simulink model "javelinSimplified"  (R2025b)
settings: Solver=VariableStepAuto  StartTime=0.0  StopTime=150  RelTol=1e-3
undefined symbols (not defined in the file): A_front, A_side, Cd_front, g, I_treghet, K_finne, Kd_altitude, Kd_pitch, Ki_altitude, Kp_altitude, Kp_pitch, L_aksial, m, rho, T, theta0, theta_dot, theta_ff, theta_ref_saturation_down, theta_ref_saturation_up, v_x0, v_z0, z0
libraries: slpidlib x2, simulink x1, SignalEditorBlockLib x1
settings Model: Creator=kristiangjestad  LastModifiedBy=kristiangjestad
settings OptimizationCC: BlockReduction=off  DefaultParameterBehavior=Inlined  BufferReuse=off

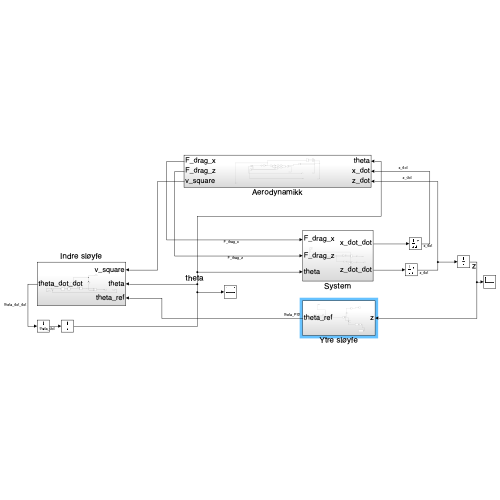
[thumbnail: Simulink's stored preview of the top-level diagram]
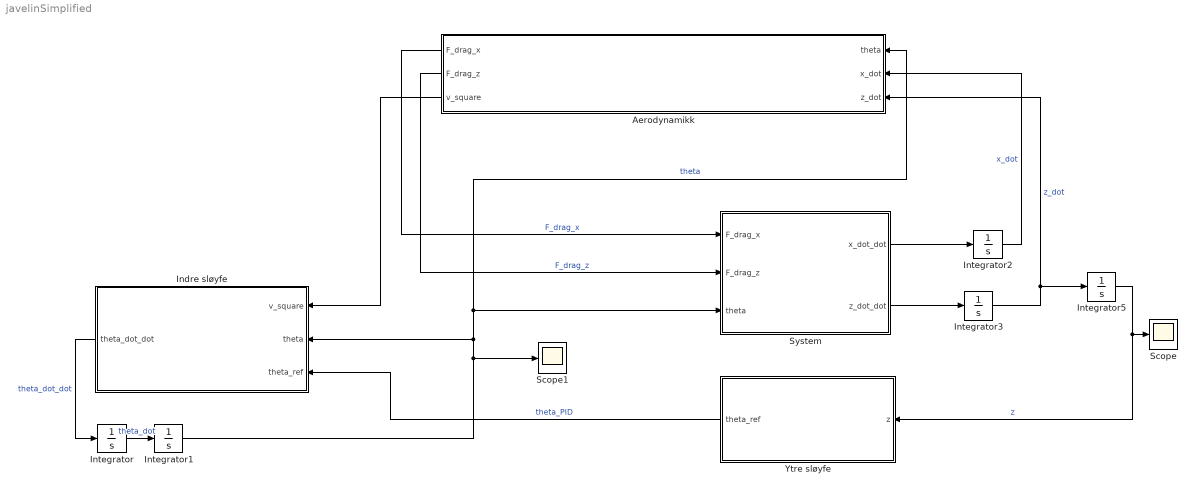
== system javelinSimplified ==
  Aerodynamikk : Subsystem
  Indre sløyfe : Subsystem
  Integrator : Integrator  InitialCondition=theta_dot
  Integrator1 : Integrator  InitialCondition=theta0
  Integrator2 : Integrator  InitialCondition=v_x0  LimitOutput=on  UpperSaturationLimit=500  LowerSaturationLimit=-0
  Integrator3 : Integrator  InitialCondition=v_z0  LimitOutput=on  UpperSaturationLimit=100  LowerSaturationLimit=-100
  Integrator5 : Integrator  InitialCondition=z0
  Scope : Scope
      settings: ActiveDisplayYMinimum=-18.802129025254686  ActiveDisplayYMaximum=169.2191612272922
  Scope1 : Scope
      settings: ActiveDisplayYMinimum=-0.013894772747961555  ActiveDisplayYMaximum=0.12049340894632314  DataLoggingVariableName=ScopeData2
  System : Subsystem
  Ytre sløyfe : Subsystem
  wires:
  Integrator3/1 -> Aerodynamikk/3(z_dot), Integrator5/1  "z_dot"
  Integrator5/1 -> Ytre sløyfe/1(z), Scope/1  "z"
  Integrator2/1 -> Aerodynamikk/2(x_dot)  "x_dot"
  Integrator/1 -> Integrator1/1  "theta_dot"
  Integrator1/1 -> Scope1/1, Aerodynamikk/1(theta), System/3(theta), Indre sløyfe/2(theta)  "theta"
  Indre sløyfe/1(theta_dot_dot) -> Integrator/1  "theta_dot_dot"
  Aerodynamikk/3(v_square) -> Indre sløyfe/1(v_square)
  Aerodynamikk/1(F_drag_x) -> System/1(F_drag_x)  "F_drag_x"
  Aerodynamikk/2(F_drag_z) -> System/2(F_drag_z)  "F_drag_z"
  System/1(x_dot_dot) -> Integrator2/1
  System/2(z_dot_dot) -> Integrator3/1
  Ytre sløyfe/1(theta_ref) -> Indre sløyfe/3(theta_ref)  "theta_PID"

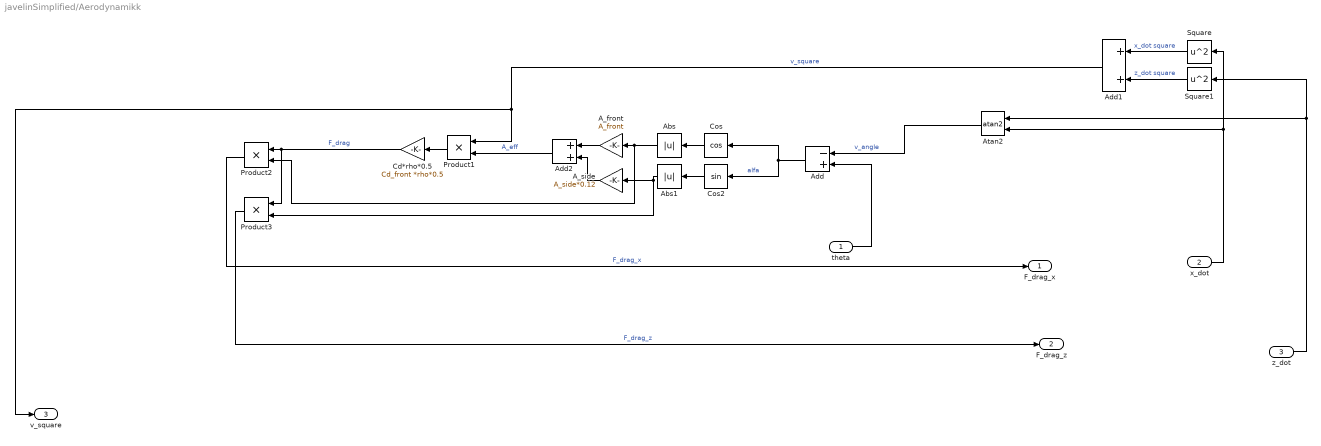
== system javelinSimplified/Aerodynamikk ==
  theta : Inport
  x_dot : Inport  Port=2
  z_dot : Inport  Port=3
  A_front : Gain  Gain=A_front
  A_side : Gain  Gain=A_side*0.12
  Abs : Abs  ZeroCross=off  SaturateOnIntegerOverflow=off
  Abs1 : Abs  ZeroCross=off  SaturateOnIntegerOverflow=off
  Add : Sum  Inputs=-+
  Add1 : Sum
  Add2 : Sum
  Atan2 : Trigonometry  Operator=atan2
  Cd*rho*0.5 : Gain  Gain=Cd_front *rho*0.5
  Cos : Trigonometry  Operator=cos
  Cos2 : Trigonometry
  Product1 : Product
  Product2 : Product
  Product3 : Product
  Square : Math  Operator=square
  Square1 : Math  Operator=square
  F_drag_x : Outport
  F_drag_z : Outport  Port=2
  v_square : Outport  Port=3
  wires:
  theta/1 -> Add/2
  Product3/1 -> F_drag_z/1  "F_drag_z"
  Square1/1 -> Add1/2  "z_dot square"
  Product1/1 -> Cd*rho*0.5/1
  z_dot/1 -> Atan2/1, Square1/1
  Cos/1 -> Abs/1
  x_dot/1 -> Atan2/2, Square/1
  A_front/1 -> Add2/1
  Abs/1 -> Product2/2, A_front/1
  Add1/1 -> v_square/1, Product1/1  "v_square"
  A_side/1 -> Add2/2
  Add2/1 -> Product1/2  "A_eff"
  Abs1/1 -> Product3/2, A_side/1
  Add/1 -> Cos2/1, Cos/1  "alfa"
  Cos2/1 -> Abs1/1
  Atan2/1 -> Add/1  "v_angle"
  Product2/1 -> F_drag_x/1  "F_drag_x"
  Square/1 -> Add1/1  "x_dot square"
  Cd*rho*0.5/1 -> Product3/1, Product2/1  "F_drag"

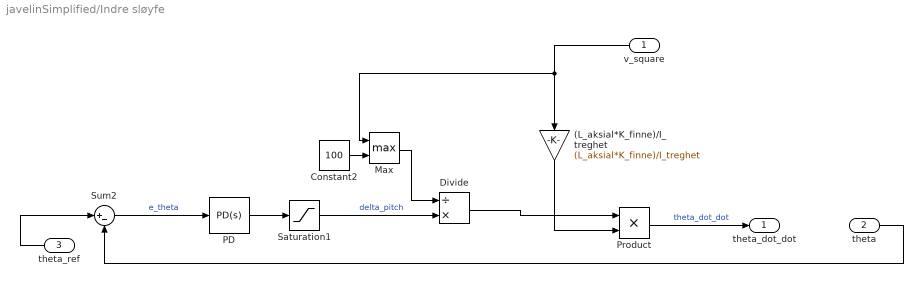
== system javelinSimplified/Indre sløyfe ==
  v_square : Inport
  theta : Inport  Port=2
  theta_ref : Inport  Port=3
  (L_aksial*K_finne)/I_treghet : Gain  Gain=(L_aksial*K_finne)/I_treghet
  Constant2 : Constant  Value=100
  Divide : Product  Inputs=/*
  Max : MinMax  Function=max  Inputs=2
  PD : slpidlib/PID Controller  Controller=PD  Form=Parallel  TimeDomain=Continuous-time  UseExternalTs=off  SampleTime=-1  IntegratorMethod=Forward Euler  FilterMethod=Forward Euler  ControllerParametersSource=internal  P=Kp_pitch  I=0  UseKiTs=off  D=Kd_pitch  UseExternalDerivativeSource=off  N=10  UseFilter=on  TunerSelectOption=Transfer Function Based (PID Tuner App)  InitialConditionSource=internal  InitialConditionForIntegrator=0  InitialConditionForFilter=0  DifferentiatorICPrevScaledInput=0  ExternalReset=none  TrackingMode=off  Kt=1  LimitOutput=on  SatLimitsSource=internal  UpperSaturationLimit=theta_ref_saturation_up  LowerSaturationLimit=theta_ref_saturation_down  LinearizeAsGain=on  AntiWindupMode=none  Kb=1  LimitIntegrator=off  UpperIntegratorSaturationLimit=inf  LowerIntegratorSaturationLimit=-inf  POutMin=[]  POutMax=[]  IOutMin=[]  IOutMax=[]  DOutMin=[]  DOutMax=[]  NOutMin=[]  NOutMax=[]  SumOutMin=[]  SumOutMax=[]  SaturationOutMin=[]  SaturationOutMax=[]  PParamMin=[]  PParamMax=[]  IParamMin=[]  IParamMax=[]  DParamMin=[]  DParamMax=[]  NParamMin=[]  NParamMax=[]  KbParamMin=[]  KbParamMax=[]  KtParamMin=[]  KtParamMax=[]  KbOutMin=[]  KbOutMax=[]  KtOutMin=[]  KtOutMax=[]  IntegratorOutMin=[]  IntegratorOutMax=[]  FilterOutMin=[]  FilterOutMax=[]  SumI1OutMin=[]  SumI1OutMax=[]  SumI2OutMin=[]  SumI2OutMax=[]  SumI3OutMin=[]  SumI3OutMax=[]  SumI4OutMin=[]  SumI4OutMax=[]  SumDOutMin=[]  SumDOutMax=[]  DifferentiatorOutMin=[]  DifferentiatorOutMax=[]  FilterDiffOutCoefMin=[]  FilterDiffOutCoefMax=[]  ReciprocalOutMin=[]  ReciprocalOutMax=[]  SumDenOutMin=[]  SumDenOutMax=[]  SumNumOutMin=[]  SumNumOutMax=[]  DivideOutMin=[]  DivideOutMax=[]  UdiffTsProdOutMin=[]  UdiffTsProdOutMax=[]  NTsProdOutMin=[]  NTsProdOutMax=[]  UintegralTsProdOutMin=[]  UintegralTsProdOutMax=[]  UngainTsProdOutMin=[]  UngainTsProdOutMax=[]  ClampingZeroOutDataTypeStr=Inherit: Inherit via back propagation  ClampingZeroOutMin=[]  ClampingZeroOutMax=[]  FilterDenConstantOutDataTypeStr=Inherit: Inherit via back propagation  FilterDenConstantOutMin=[]  FilterDenConstantOutMax=[]  PCopyOutDataTypeStr=Inherit: Inherit via back propagation  PCopyOutMin=[]  PCopyOutMax=[]  NCopyOutDataTypeStr=Inherit: Inherit via back propagation  NCopyOutMin=[]  NCopyOutMax=[]  IntegratorContinuousStateAttributes=''  IntegratorStateMustResolveToSignalObject=off  IntegratorRTWStateStorageClass=Auto  FilterContinuousStateAttributes=''  FilterStateMustResolveToSignalObject=off  FilterRTWStateStorageClass=Auto  ParallelPVariant=InternalParameters  IdealPVariant=Disabled  IVariant=Disabled  DVariant=InternalParameters  IntegratorVariant=Disabled  SatVariant=Enabled  AWVariant=Disabled  PCopyVariant=Disabled  TRVariant=Disabled  FdbkBlocksVariant=Forward  IdealPFdbkVariant=Disabled  SatFdbkVariant=Disabled  DerivativeFilterVariant=ContFilter  NVariant=InternalParameters  NCopyVariant=Disabled  FilterICVariant=InternalICsFilter  IntegratorICVariant=Disabled  ExternalResetVariant=Disabled  TRSumVariant=Passthrough  SumFdbkVariant=Disabled  SumVariant=Sum_PD  TsampFilterVariant=InternalTs  TsampNgainVariant=Passthrough  TsampIntegralVariant=Disabled_SignalSpec  ExternalSaturationOutDataTypeStr=Inherit: Same as second input  DerivativeSourceVariant=ErrorSignal  PreIntVariant=InternalPreInt
  Product : Product
  Saturation1 : Saturate  UpperLimit=theta_ref_saturation_up  LowerLimit=theta_ref_saturation_down  ZeroCross=off
  Sum2 : Sum  Inputs=|+-
  theta_dot_dot : Outport
  wires:
  theta_ref/1 -> Sum2/1
  Max/1 -> Divide/1
  Product/1 -> theta_dot_dot/1  "theta_dot_dot"
  theta/1 -> Sum2/2
  (L_aksial*K_finne)/I_treghet/1 -> Product/2
  v_square/1 -> Max/1, (L_aksial*K_finne)/I_treghet/1
  PD/1 -> Saturation1/1
  Sum2/1 -> PD/1  "e_theta"
  Constant2/1 -> Max/2
  Divide/1 -> Product/1
  Saturation1/1 -> Divide/2  "delta_pitch"

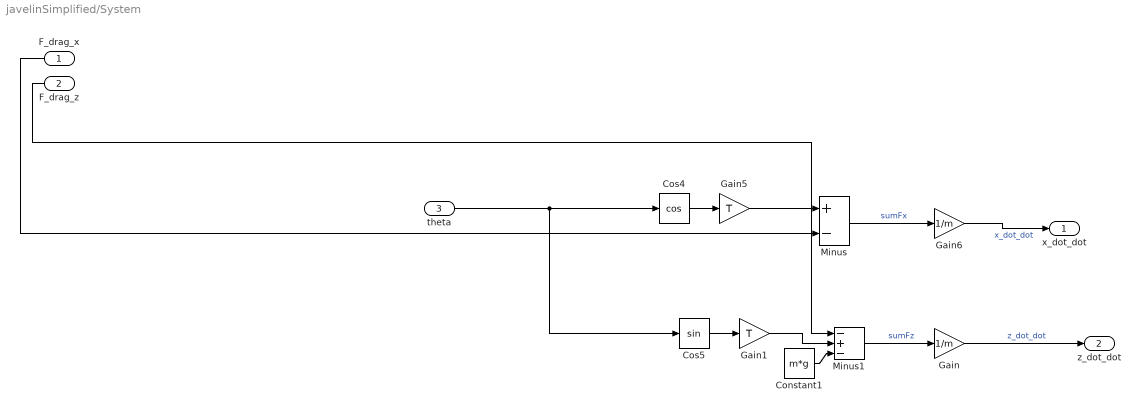
== system javelinSimplified/System ==
  F_drag_x : Inport
  F_drag_z : Inport  Port=2
  theta : Inport  Port=3
  Constant1 : Constant  Value=m*g
  Cos4 : Trigonometry  Operator=cos
  Cos5 : Trigonometry
  Gain : Gain  Gain=1/m
  Gain1 : Gain  Gain=T
  Gain5 : Gain  Gain=T
  Gain6 : Gain  Gain=1/m
  Minus : Sum  Inputs=+-
  Minus1 : Sum  Inputs=-+-
  x_dot_dot : Outport
  z_dot_dot : Outport  Port=2
  wires:
  Gain6/1 -> x_dot_dot/1  "x_dot_dot"
  Gain5/1 -> Minus/1
  theta/1 -> Cos5/1, Cos4/1
  F_drag_x/1 -> Minus/2
  F_drag_z/1 -> Minus1/1
  Minus/1 -> Gain6/1  "sumFx"
  Constant1/1 -> Minus1/3
  Gain/1 -> z_dot_dot/1  "z_dot_dot"
  Cos4/1 -> Gain5/1
  Cos5/1 -> Gain1/1
  Gain1/1 -> Minus1/2
  Minus1/1 -> Gain/1  "sumFz"

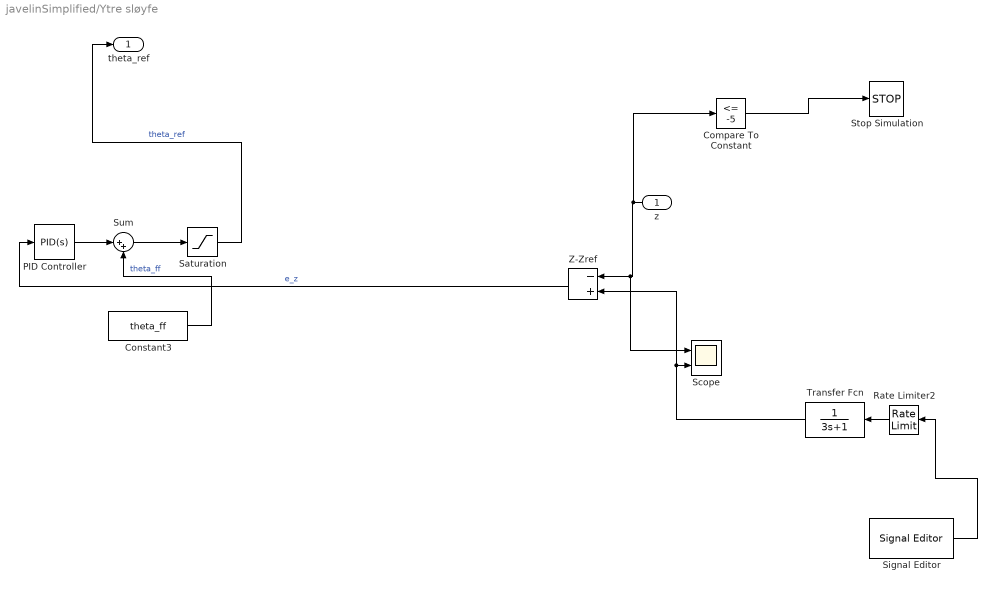
== system javelinSimplified/Ytre sløyfe ==
  z : Inport
  Compare To Constant : simulink/Logic and Bit Operations/Compare To Constant  relop=<=  const=-5  OutDataTypeStr=boolean
  Constant3 : Constant  Value=theta_ff
  PID Controller : slpidlib/PID Controller  Controller=PID  Form=Parallel  TimeDomain=Continuous-time  UseExternalTs=off  SampleTime=-1  IntegratorMethod=Forward Euler  FilterMethod=Forward Euler  ControllerParametersSource=internal  P=Kp_altitude  I=Ki_altitude  UseKiTs=off  D=Kd_altitude  UseExternalDerivativeSource=off  N=100  UseFilter=on  TunerSelectOption=Transfer Function Based (PID Tuner App)  InitialConditionSource=internal  InitialConditionForIntegrator=0  InitialConditionForFilter=0  DifferentiatorICPrevScaledInput=0  ExternalReset=none  TrackingMode=off  Kt=1  LimitOutput=on  SatLimitsSource=internal  UpperSaturationLimit=theta_ref_saturation_up  LowerSaturationLimit=theta_ref_saturation_down  LinearizeAsGain=on  AntiWindupMode=clamping  Kb=1  LimitIntegrator=off  UpperIntegratorSaturationLimit=inf  LowerIntegratorSaturationLimit=-inf  POutMin=[]  POutMax=[]  IOutMin=[]  IOutMax=[]  DOutMin=[]  DOutMax=[]  NOutMin=[]  NOutMax=[]  SumOutMin=[]  SumOutMax=[]  SaturationOutMin=[]  SaturationOutMax=[]  PParamMin=[]  PParamMax=[]  IParamMin=[]  IParamMax=[]  DParamMin=[]  DParamMax=[]  NParamMin=[]  NParamMax=[]  KbParamMin=[]  KbParamMax=[]  KtParamMin=[]  KtParamMax=[]  KbOutMin=[]  KbOutMax=[]  KtOutMin=[]  KtOutMax=[]  IntegratorOutMin=[]  IntegratorOutMax=[]  FilterOutMin=[]  FilterOutMax=[]  SumI1OutMin=[]  SumI1OutMax=[]  SumI2OutMin=[]  SumI2OutMax=[]  SumI3OutMin=[]  SumI3OutMax=[]  SumI4OutMin=[]  SumI4OutMax=[]  SumDOutMin=[]  SumDOutMax=[]  DifferentiatorOutMin=[]  DifferentiatorOutMax=[]  FilterDiffOutCoefMin=[]  FilterDiffOutCoefMax=[]  ReciprocalOutMin=[]  ReciprocalOutMax=[]  SumDenOutMin=[]  SumDenOutMax=[]  SumNumOutMin=[]  SumNumOutMax=[]  DivideOutMin=[]  DivideOutMax=[]  UdiffTsProdOutMin=[]  UdiffTsProdOutMax=[]  NTsProdOutMin=[]  NTsProdOutMax=[]  UintegralTsProdOutMin=[]  UintegralTsProdOutMax=[]  UngainTsProdOutMin=[]  UngainTsProdOutMax=[]  ClampingZeroOutDataTypeStr=Inherit: Inherit via back propagation  ClampingZeroOutMin=[]  ClampingZeroOutMax=[]  FilterDenConstantOutDataTypeStr=Inherit: Inherit via back propagation  FilterDenConstantOutMin=[]  FilterDenConstantOutMax=[]  PCopyOutDataTypeStr=Inherit: Inherit via back propagation  PCopyOutMin=[]  PCopyOutMax=[]  NCopyOutDataTypeStr=Inherit: Inherit via back propagation  NCopyOutMin=[]  NCopyOutMax=[]  IntegratorContinuousStateAttributes=''  IntegratorStateMustResolveToSignalObject=off  IntegratorRTWStateStorageClass=Auto  FilterContinuousStateAttributes=''  FilterStateMustResolveToSignalObject=off  FilterRTWStateStorageClass=Auto  ParallelPVariant=InternalParameters  IdealPVariant=Disabled  IVariant=InternalParameters  DVariant=InternalParameters  IntegratorVariant=Continuous  SatVariant=Enabled  AWVariant=ContClampingParallel  PCopyVariant=Disabled  TRVariant=Disabled  FdbkBlocksVariant=Forward  IdealPFdbkVariant=Disabled  SatFdbkVariant=Disabled  DerivativeFilterVariant=ContFilter  NVariant=InternalParameters  NCopyVariant=Disabled  FilterICVariant=InternalICsFilter  IntegratorICVariant=InternalICs  ExternalResetVariant=Disabled  TRSumVariant=Passthrough  SumFdbkVariant=Disabled  SumVariant=Sum_PID  TsampFilterVariant=InternalTs  TsampNgainVariant=Passthrough  TsampIntegralVariant=Disabled_SignalSpec  ExternalSaturationOutDataTypeStr=Inherit: Same as second input  DerivativeSourceVariant=ErrorSignal  PreIntVariant=InternalPreInt
  Rate Limiter2 : RateLimiter  RisingSlewLimit=10  FallingSlewLimit=-20
  Saturation : Saturate  UpperLimit=theta_ref_saturation_up  LowerLimit=theta_ref_saturation_down  ZeroCross=off
  Scope : Scope  NumInputPorts=2
      settings: ActiveDisplayYMinimum=-20.704780798477266  ActiveDisplayYMaximum=186.34302718629542
  Signal Editor : SignalEditorBlockLib/Signal Editor  FileName=/Users/kristiangjestad/ntnu/ttk4105/javelin/matlab/data/bane.mat  ActiveScenario=Scenario  ActiveSignal=Signal 1  IsBus=off  OutputBusObjectStr=Bus: BusObject  SampleTime=0  ZeroCross=off  OutputAfterFinalValue=Setting to zero  Unit=inherit  PreserveSignalName=on  ApplySigPropsToAllScenarios=on  ApplySigPropsToAllSignals=off  SignalPropertySource=Dialog parameters
  Stop Simulation : Stop
  Sum : Sum  Inputs=|++
  Transfer Fcn : TransferFcn  Denominator=[3 1]
  Z-Zref : Sum  Inputs=-+
  theta_ref : Outport
  wires:
  Sum/1 -> Saturation/1
  Saturation/1 -> theta_ref/1  "theta_ref"
  PID Controller/1 -> Sum/1
  Constant3/1 -> Sum/2  "theta_ff"
  Z-Zref/1 -> PID Controller/1  "e_z"
  z/1 -> Compare To Constant/1, Scope/1, Z-Zref/1
  Rate Limiter2/1 -> Transfer Fcn/1
  Signal Editor/1 -> Rate Limiter2/1
  Compare To Constant/1 -> Stop Simulation/1
  Transfer Fcn/1 -> Z-Zref/2, Scope/2
